simulink model "Demo1_final"  (R2015a)
settings: Solver=ode45  StartTime=0.0  StopTime=inf  RelTol=1e-3
InitFcn:
  | Initilization_simulink
values from neighbouring files (symbols this model uses):
  field_x = sqrt(field_x_vec(1)^2 + field_x_vec(2)^2)    [CalibrateField.m]    (also in Config.mat = 11.7868563762)
  field_y = sqrt(field_y_vec(1)^2 + field_y_vec(2)^2)    [CalibrateField.m]    (also in Config.mat = 8.01974905199)
  items = [CR1;CR2;CR3;CR4]    [CalibrateField.m]    (also in Config.mat = [-6.14339468658  -3.99467558804; 5.6178847579  -4.007837403;)
  ref = [3.07784055213  -4.49067034415  0; -3.25612463225  -4.14482557696  0; 3.15604151052  4.41744641428  0]    [Config.mat]
  thetaCamX = 43*pi/180    (= 0.750491578358)    [Initilization_simulink.m]    (also in debugging_refereeing.m = 1.01229096616)
  thetaCamY = 32*pi/180    (= 0.558505360638)    [Initilization_simulink.m]
undefined symbols (not defined in the file or in its folder): backim, drone1
libraries: visionsinks x2
settings Model: CovSFcnEnable=off  Creator=tzwijger  LastModifiedBy=tzwijger
settings DebuggingCC: SolverPrmCheckMsg=warning

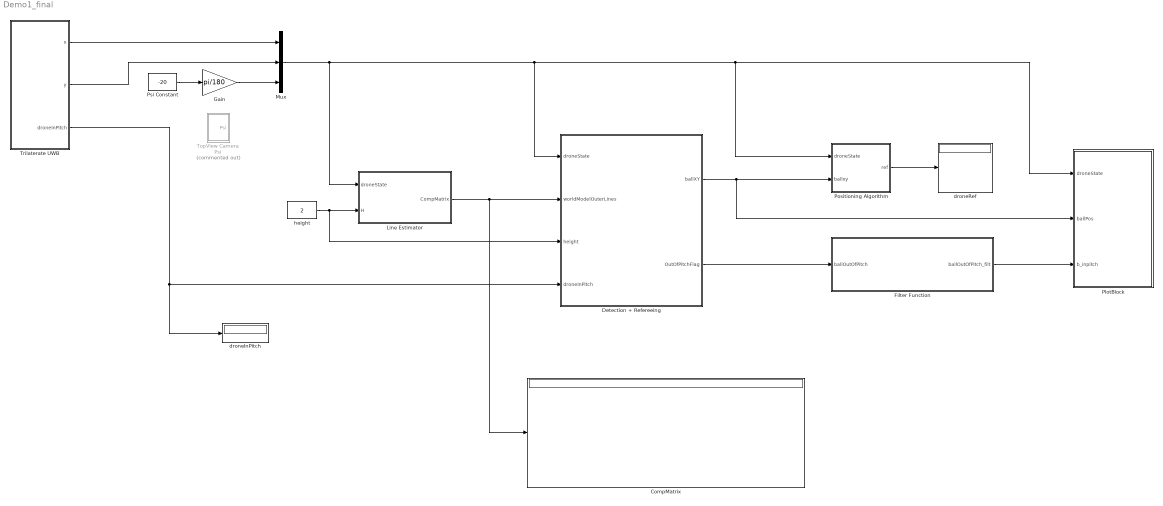
== system Demo1_final ==
  CompMatrix : Display
  Detection + Refereeing : Subsystem
  Filter Function : MATLAB Function  TreatAsAtomicUnit=on
  Gain : Gain  Gain=pi/180
  Line Estimator : Subsystem
  Mux : Mux  Inputs=3
  PlotBlock : Subsystem
  Positioning Algorithm : Subsystem
  Psi Constant : Constant  Value=-20
  TopView Camera Psi : Subsystem  Commented=on
  Trilaterate UWB : Subsystem
  droneInPitch : Display
  droneRef : Display
  height : Constant  Value=2
  wires:
  Line Estimator/1(CompMatrix) -> Detection + Refereeing/2(worldModelOuterLines), CompMatrix/1
  Trilaterate UWB/3(droneInPitch) -> droneInPitch/1, Detection + Refereeing/4(droneInPitch)
  height/1 -> Detection + Refereeing/3(height), Line Estimator/2(H)
  Mux/1 -> Line Estimator/1(droneState), Detection + Refereeing/1(droneState), Positioning Algorithm/1(droneState), PlotBlock/1(droneState)
  Detection + Refereeing/1(ballXY) -> PlotBlock/2(ballPos), Positioning Algorithm/2(ballxy)
  Positioning Algorithm/1(ref) -> droneRef/1
  Trilaterate UWB/1(x) -> Mux/1
  Trilaterate UWB/2(y) -> Mux/2
  Detection + Refereeing/2(OutOfPitchFlag) -> Filter Function/1(ballOutOfPitch)
  Filter Function/1(ballOutOfPitch_filt) -> PlotBlock/3(b_inpitch)
  Psi Constant/1 -> Gain/1
  Gain/1 -> Mux/3

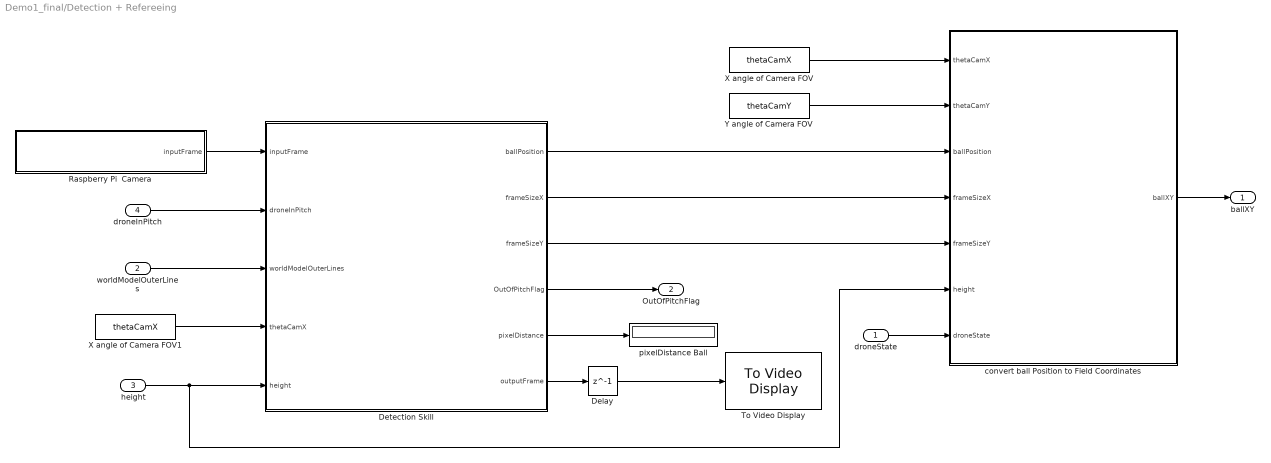
== system Demo1_final/Detection + Refereeing ==
  droneState : Inport
  worldModelOuterLines : Inport  Port=2
  height : Inport  Port=3
  droneInPitch : Inport  Port=4
  Delay : Delay  DelayLength=1  SampleTime=0.25
  Detection Skill : MATLAB Function  TreatAsAtomicUnit=on
  Raspberry Pi  Camera : MATLAB Function  TreatAsAtomicUnit=on
  To Video Display : visionsinks/To Video Display  windowSizeMode=True size (1:1)  openAtMdlStart=on  fullScreen=off  videoWindowX=54  videoWindowY=328  saveWindowSize=off  videoWindowWidth=320  videoWindowHeight=240  inputColorFormat=RGB  inputType=Obsolete  imagePorts=One multidimensional signal  OutputDevice=On-screen video monitor  dataOrg=Column-major  isWindowOpen=off
  X angle of Camera FOV : Constant  Value=thetaCamX
  X angle of Camera FOV1 : Constant  Value=thetaCamX
  Y angle of Camera FOV : Constant  Value=thetaCamY
  convert ball Position to Field Coordinates : Subsystem
  pixelDistance Ball : Display
  ballXY : Outport
  OutOfPitchFlag : Outport  Port=2
  wires:
  droneState/1 -> convert ball Position to Field Coordinates/7(droneState)
  convert ball Position to Field Coordinates/1(ballXY) -> ballXY/1
  X angle of Camera FOV/1 -> convert ball Position to Field Coordinates/1(thetaCamX)
  Y angle of Camera FOV/1 -> convert ball Position to Field Coordinates/2(thetaCamY)
  height/1 -> convert ball Position to Field Coordinates/6(height), Detection Skill/5(height)
  X angle of Camera FOV1/1 -> Detection Skill/4(thetaCamX)
  worldModelOuterLines/1 -> Detection Skill/3(worldModelOuterLines)
  droneInPitch/1 -> Detection Skill/2(droneInPitch)
  Raspberry Pi  Camera/1(inputFrame) -> Detection Skill/1(inputFrame)
  Detection Skill/5(pixelDistance) -> pixelDistance Ball/1
  Detection Skill/4(OutOfPitchFlag) -> OutOfPitchFlag/1
  Detection Skill/1(ballPosition) -> convert ball Position to Field Coordinates/3(ballPosition)
  Detection Skill/2(frameSizeX) -> convert ball Position to Field Coordinates/4(frameSizeX)
  Detection Skill/3(frameSizeY) -> convert ball Position to Field Coordinates/5(frameSizeY)
  Detection Skill/6(outputFrame) -> Delay/1
  Delay/1 -> To Video Display/1

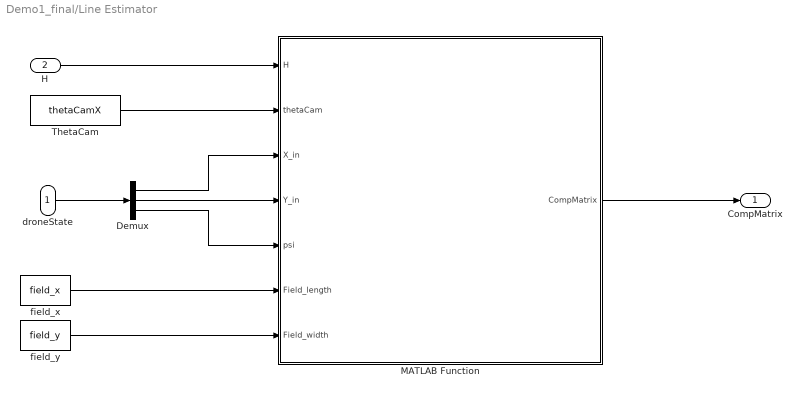
== system Demo1_final/Line Estimator ==
  droneState : Inport
  H : Inport  Port=2
  Demux : Demux  Outputs=3
  MATLAB Function : MATLAB Function  TreatAsAtomicUnit=on
  ThetaCam : Constant  Value=thetaCamX
  field_x : Constant  Value=field_x
  field_y : Constant  Value=field_y
  CompMatrix : Outport
  wires:
  MATLAB Function/1(CompMatrix) -> CompMatrix/1
  ThetaCam/1 -> MATLAB Function/2(thetaCam)
  H/1 -> MATLAB Function/1(H)
  droneState/1 -> Demux/1
  field_x/1 -> MATLAB Function/6(Field_length)
  field_y/1 -> MATLAB Function/7(Field_width)
  Demux/1 -> MATLAB Function/3(X_in)
  Demux/2 -> MATLAB Function/4(Y_in)
  Demux/3 -> MATLAB Function/5(psi)

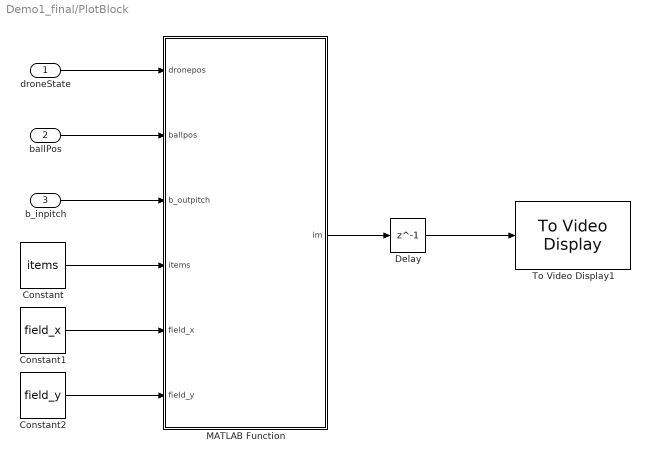
== system Demo1_final/PlotBlock ==
  droneState : Inport
  ballPos : Inport  Port=2
  b_inpitch : Inport  Port=3
  Constant : Constant  Value=items
  Constant1 : Constant  Value=field_x
  Constant2 : Constant  Value=field_y
  Delay : Delay  DelayLength=1  SampleTime=0.25
  MATLAB Function : MATLAB Function  TreatAsAtomicUnit=on
  To Video Display1 : visionsinks/To Video Display  windowSizeMode=True size (1:1)  openAtMdlStart=on  fullScreen=off  videoWindowX=559  videoWindowY=31  saveWindowSize=off  videoWindowWidth=883  videoWindowHeight=607  inputColorFormat=RGB  inputType=Obsolete  imagePorts=One multidimensional signal  OutputDevice=On-screen video monitor  dataOrg=Column-major  isWindowOpen=off
  wires:
  Constant/1 -> MATLAB Function/4(items)
  ballPos/1 -> MATLAB Function/2(ballpos)
  droneState/1 -> MATLAB Function/1(dronepos)
  Constant1/1 -> MATLAB Function/5(field_x)
  Constant2/1 -> MATLAB Function/6(field_y)
  MATLAB Function/1(im) -> Delay/1
  Delay/1 -> To Video Display1/1
  b_inpitch/1 -> MATLAB Function/3(b_outpitch)

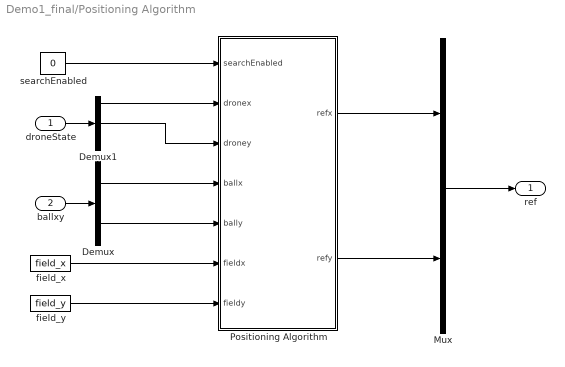
== system Demo1_final/Positioning Algorithm ==
  droneState : Inport
  ballxy : Inport  Port=2
  Demux : Demux  Outputs=2
  Demux1 : Demux  Outputs=3
  Mux : Mux  Inputs=2
  Positioning Algorithm : MATLAB Function  TreatAsAtomicUnit=on
  field_x : Constant  Value=field_x
  field_y : Constant  Value=field_y
  searchEnabled : Constant  Value=0
  ref : Outport
  wires:
  Demux/2 -> Positioning Algorithm/5(bally)
  Demux/1 -> Positioning Algorithm/4(ballx)
  Positioning Algorithm/1(refx) -> Mux/1
  Positioning Algorithm/2(refy) -> Mux/2
  Mux/1 -> ref/1
  field_x/1 -> Positioning Algorithm/6(fieldx)
  field_y/1 -> Positioning Algorithm/7(fieldy)
  droneState/1 -> Demux1/1
  Demux1/1 -> Positioning Algorithm/2(dronex)
  ballxy/1 -> Demux/1
  Demux1/2 -> Positioning Algorithm/3(droney)
  searchEnabled/1 -> Positioning Algorithm/1(searchEnabled)

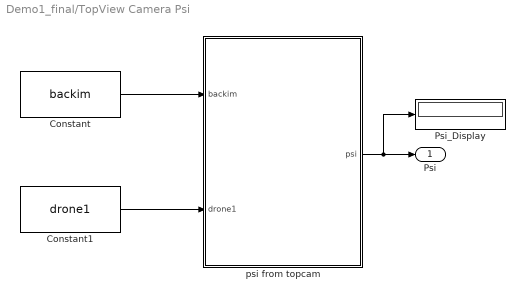
== system Demo1_final/TopView Camera Psi ==
  Constant : Constant  Value=backim
  Constant1 : Constant  Value=drone1
  Psi_Display : Display
  psi from topcam : MATLAB Function  TreatAsAtomicUnit=on
  Psi : Outport
  wires:
  Constant1/1 -> psi from topcam/2(drone1)
  Constant/1 -> psi from topcam/1(backim)
  psi from topcam/1(psi) -> Psi_Display/1, Psi/1

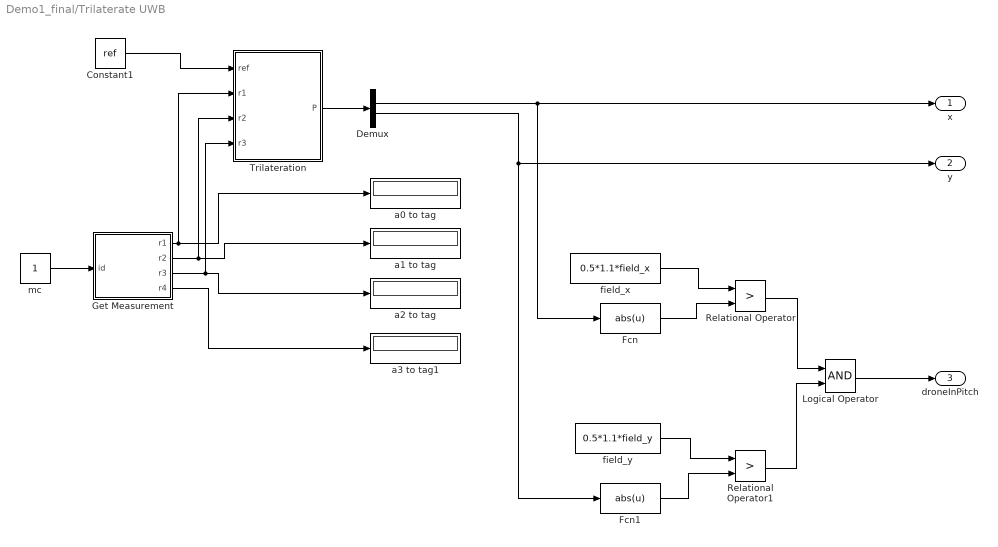
== system Demo1_final/Trilaterate UWB ==
  Constant1 : Constant  Value=ref
  Demux : Demux
  Fcn : Fcn  Expr=abs(u)
  Fcn1 : Fcn  Expr=abs(u)
  Get Measurement : MATLAB Function  TreatAsAtomicUnit=on
  Logical Operator : Logic  AllPortsSameDT=off  OutDataTypeStr=boolean
  Relational Operator : RelationalOperator  Operator=>  OutDataTypeStr=boolean
  Relational Operator1 : RelationalOperator  Operator=>  OutDataTypeStr=boolean
  Trilateration : MATLAB Function  TreatAsAtomicUnit=on
  a0 to tag : Display
  a1 to tag : Display
  a2 to tag : Display
  a3 to tag1 : Display
  field_x : Constant  Value=0.5*1.1*field_x
  field_y : Constant  Value=0.5*1.1*field_y
  mc : Constant
  x : Outport
  y : Outport  Port=2
  droneInPitch : Outport  Port=3
  wires:
  Demux/3 -> Fcn1/1, y/1
  Demux/2 -> Fcn/1, x/1
  Trilateration/1(P) -> Demux/1
  Constant1/1 -> Trilateration/1(ref)
  Get Measurement/3(r3) -> a2 to tag/1, Trilateration/4(r3)
  Get Measurement/2(r2) -> a1 to tag/1, Trilateration/3(r2)
  mc/1 -> Get Measurement/1(id)
  Get Measurement/1(r1) -> Trilateration/2(r1), a0 to tag/1
  Get Measurement/4(r4) -> a3 to tag1/1
  Fcn/1 -> Relational Operator/2
  field_x/1 -> Relational Operator/1
  field_y/1 -> Relational Operator1/1
  Fcn1/1 -> Relational Operator1/2
  Relational Operator1/1 -> Logical Operator/2
  Relational Operator/1 -> Logical Operator/1
  Logical Operator/1 -> droneInPitch/1

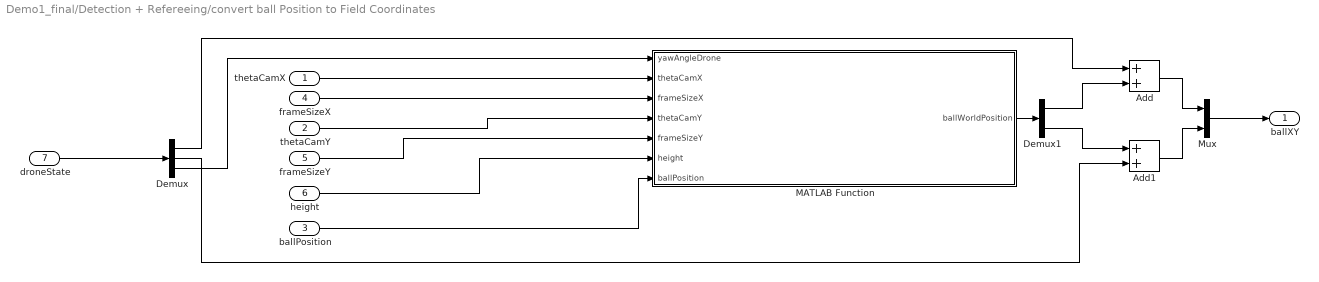
== system Demo1_final/Detection + Refereeing/convert ball Position to Field Coordinates ==
  thetaCamX : Inport
  thetaCamY : Inport  Port=2
  ballPosition : Inport  Port=3
  frameSizeX : Inport  Port=4
  frameSizeY : Inport  Port=5
  height : Inport  Port=6
  droneState : Inport  Port=7
  Add : Sum
  Add1 : Sum
  Demux : Demux  Outputs=3
  Demux1 : Demux  Outputs=2
  MATLAB Function : MATLAB Function  TreatAsAtomicUnit=on
  Mux : Mux  Inputs=2
  ballXY : Outport
  wires:
  thetaCamY/1 -> MATLAB Function/4(thetaCamY)
  height/1 -> MATLAB Function/6(height)
  thetaCamX/1 -> MATLAB Function/2(thetaCamX)
  ballPosition/1 -> MATLAB Function/7(ballPosition)
  frameSizeY/1 -> MATLAB Function/5(frameSizeY)
  Mux/1 -> ballXY/1
  Add/1 -> Mux/1
  Add1/1 -> Mux/2
  MATLAB Function/1(ballWorldPosition) -> Demux1/1
  frameSizeX/1 -> MATLAB Function/3(frameSizeX)
  Demux/1 -> Add/1
  Demux1/2 -> Add1/1
  Demux1/1 -> Add/2
  droneState/1 -> Demux/1
  Demux/3 -> MATLAB Function/1(yawAngleDrone)
  Demux/2 -> Add1/2

== matlab function Demo1_final/Trilaterate UWB/Trilateration ==
  data: P output; ref input; r1 input; r2 input; r3 input
function P  = trilateration(ref,r1,r2,r3)%,fign,field2im_params)
% persistent plots k nrplots

coder.extrinsic('Trilateration')

% if isempty(plots)
%     plots = [0];
%     k = 1;
%     nrplots = 10;
% end

P = zeros(4,1);
P = Trilateration(ref',[r1 r2 r3],eye(3));

% % Plot and print results
% [plots, k] = update_plot_trilat(plots, k, fign, P(2:3), field2im_params, nrplots);

== matlab function Demo1_final/Trilaterate UWB/Get Measurement ==
  data: id input; r1 output; r2 output; r3 output; r4 output
function [r1,r2,r3,r4] = GetMC_sm(id) 
    % Input: Serial Port to A0
    %        
    % Output: Raw data for triangulation
    %
    % Message syntax is explained in the Decawave documentation
    % DecaRangeRTLS_PC_Source_Code_Guide.pdf  - Section 2.3.2
    % DecaRangeRTLS_ARM_Source_Code_Guide.pdf - Section 2.6

    % Make sure to get a measurement with the correct identifier
    persistent s count;
    %coder.extrinsic('instrfind','delete','serial','fscanf','strsplit')
    coder.extrinsic('instrfind','delete','serial','fscanf','GetMC','flushinput')
    
    r1 = 0; r2 = 0; r3 = 0; r4 = 0;
    
    if isempty(s)
        ports = instrfind;
        if ~isempty(ports)
            fclose(ports);
            delete(ports);
        end
        % Establish new connection
        s = serial('COM33','BaudRate',9600,'Parity','None');

        % Open connection
        fopen(s);
        fscanf(s); % Get init mc out of the way and test connection
        
        count = 0;
    end
    
    ids = ['mc';'mr';'ma'];
    id = ids(id,:);
    
    dist = zeros(1,4);
    
    dist = GetMC(s,id);
    r1 = dist(1);
    r2 = dist(2);
    r3 = dist(3);
    r4 = dist(4); 
    
    if count > 10
        % We are reading values slower than they come in
        % Sometimes the buffer needs to be cleared
        flushinput(s)
        count = 0;
    else
        count = count + 1;
    end
end

== matlab function Demo1_final/Line Estimator/MATLAB Function ==
  data: H input; CompMatrix output; thetaCam input; X_in input; Y_in input; psi input; Field_length input; Field_width input
function CompMatrix   = World(H,thetaCam,X_in,Y_in,psi,Field_length,Field_width)

% %field line numbering:  222222222222222222223
%                         1                   3
%                         1                   3
%                         1                   3
%                         1                   3
%                         1                   3
%                         144444444444444444443

% Psi: conter-clock wise positive. zero at localization Y axis
% Theta and rho are defined according to matlab hough transform matrix

Vision=2*H*tan(thetaCam/2);

X_Vision=Vision;  %<--------------->
% Y_Vision=Vision*(480/640);  %|
                            %|

% Lvision=sqrt((X_Vision^2)+(Y_Vision^2));
% init_angel=atan(640/480);
% X=X_in-(Lvision/2)*sin(init_angel-psi);  %moving the origin from center of the camera to top left
% Y=Y_in+(Lvision/2)*cos(init_angel-psi);
%%%%%%%%%%%%%%%%%%%%%%%%%%%%%%%%%%%%%%%%%%%%%%%%%%%%%%%%%%%%%%%%%%%%%%%%%%
%Field_length=10;   %dimentions of the field%<--------------->

%Field_width=8; %|
                %|

pixelDistanceWorld=(H*tan(thetaCam/2))/(320/2);
Rx2=rotx(-180);
Rz2=rotz(psi*180/pi);
P2=[-320/2*pixelDistanceWorld;-240/2*pixelDistanceWorld; 0];
P3=Rx2*Rz2*P2;
P4=[X_in+P3(1) Y_in+P3(2)];
                
%%%%%%%%%%%%%%%%%%%%%%%%%%%%%%%%%%%%%%%%%%%%%%%%%%%%%%%%%%%%%%%%%%%%%%%%%%%
rho1=abs(P4(1)+(Field_length)/2); %calculate rho of each side line with respect to top left cordinate
rho2=abs(-P4(2)+(Field_width)/2);
rho3= abs(-P4(1)+(Field_length)/2);
rho4= abs(P4(2)+(Field_width)/2);
%%%%%%%%%%%%%%%%%%%%%%%%%%%%%%%%%%%%%%%%%%%%%%%%%%%%%%%%%%%%%%%%%%%%%%%%
X1=X_in;  %having center to compare the distance and rho
Y1=Y_in;

rho11=abs(X1+(Field_length)/2);
rho21=abs(-Y1+(Field_width)/2);
rho31= abs(-X1+(Field_length)/2);
rho41= abs(Y1+(Field_width)/2);



%%%%%%%%%%%%%%%%%%%%%%%%%%%%%%%%%%%%%%%%%%%%%%%%%%%%%%%%%%%%%%%%%%%%%%%%%%
theta1=(pi)-psi;       %calculate the theta of each side line
theta2=(-pi/2)-psi;
theta3=(0)-psi;
theta4=(pi/2)-psi;
%%%%%%%%%%%%%%%%%%%%%%%%%%%%%%%%%%%%%%%%%%%%%%%%%%%%%%%%%%%%%%%%%%%%%%%%%%

Lines=[rho1,theta1,rho11;
rho2,theta2,rho21;
rho3,theta3,rho31;
rho4,theta4,rho41];
B=zeros(4,5);



for k=1:4
    
    i=0;
    rho=Lines(k,1);
    theta=Lines(k,2);
    %if -Y_Vision*sin(theta)<rho &&  rho<X_Vision*cos(theta)
    if Lines(k,3)<X_Vision/2
        i=1;
        

    end
    while theta>=(2*pi) 
        theta=theta-2*pi;
    end
    while theta<0
        theta=theta+2*pi;
    end
    
        while theta>=(pi/2) 
        theta=theta-pi;
    end
    while theta<-pi/2
        theta=theta+pi;
    end
    
    B(k,:)=[k i 0 rho theta];
end
B(1,3)=2;
B(2,3)=1;
B(3,3)=2;
B(4,3)=1;

CompMatrix=zeros(4,5);
CompMatrix=B;

== matlab function Demo1_final/Detection + Refereeing/Detection Skill ==
  data: inputFrame input; droneInPitch input; worldModelOuterLines input; thetaCamX input; height input; ballPosition output; frameSizeX output; frameSizeY output; OutOfPitchFlag output; pixelDistance output; outputFrame output
% Author: Nestor Hernandez Rodriguez
% Last Update: 9-03-2016
% Technical University of Eindhoven
% Mechatronic Systems Design PDEng trainee

function [ballPosition,...
          frameSizeX,...
          frameSizeY,...
          OutOfPitchFlag,...
          pixelDistance,...
          outputFrame] = detectionSkillAndRefereeing(...
                                                    inputFrame,...
                                                    droneInPitch,...
                                                    worldModelOuterLines,...
                                                    thetaCamX,...
                                                    height)
                                                 
    coder.extrinsic('detectionSkill','refereeingOutOfPitch','imresize')
    
    % Prepare outputs detection skill
    ballPosition = zeros(1,2);
    %selectedLines = zeros(50,2);
    ballStatusFlag = 0;
    lineStatusFlag = 0;
    %inputFrame = imresize(inputFrame,0.65,'bilinear');
    
    outputFrame = uint8(zeros(size(inputFrame)));
    
    % Prepare outputs Refereeing function
    OutOfPitchFlag = 0;
%     selectedFilteredLines = zeros(2,6);
    pixelDistance=0;
    
    % Prepare constant/unused inputs Refereeing function
    numOutOfBoundLines = 0;
    numOutOfBoundLines = sum(worldModelOuterLines(:,2));
    
    % Prepare Other Inputs
    temp = size(inputFrame);
    frameSizeX = temp(2);
    frameSizeY = temp(1);
    frameProperties = [frameSizeY frameSizeX];
    if sum(worldModelOuterLines(:,2)) > 0
        lineDetectionEnabled = 1;
    else
        lineDetectionEnabled = 0; 
    end
    
    [ballPosition,... 
     selectedLines,... 
     outputFrame] = detectionSkill(lineDetectionEnabled,...
                                   inputFrame);
                               
    selectedLines                                                             
    [OutOfPitchFlag,...
        pixelDistance]= refereeingOutOfPitch(...
                                           ballPosition,...
                                           selectedLines,...
                                           numOutOfBoundLines,...
                                           frameProperties,...
                                           droneInPitch,...
                                           thetaCamX,...
                                           height,...                                           
                                           worldModelOuterLines);
end

== matlab function Demo1_final/TopView Camera Psi/psi from topcam ==
  data: backim input; psi output; drone1 input
function psi = fcn(backim, drone1)
%% get psi angle from top camera
% this function is the improcdrones.m implemented for ONLY ONE DRONE and 
% therefore reduced.




coder.extrinsic('psi_topviewcam_wrapped')
    
    psi = 0;
    psi = psi_topviewcam_wrapped(backim, drone1);

end

== matlab function Demo1_final/Positioning Algorithm/Positioning Algorithm ==
  data: searchEnabled input; dronex input; droney input; ballx input; refx output; bally input; refy output; fieldx input; fieldy input
function [refx,refy] = positionDrone(searchEnabled,dronex,droney,ballx,bally,fieldx,fieldy)
% ball position [-999 -999] -> No Ball Position Known
    persistent searchArray count step
    if isempty(searchArray)
       count = 1;
       i = 1;
       step = 1;
       searchArray = zeros(100,2);% Size HAS to be predetermined (...Simulink...)
       for y = -0.5*fieldy:step:0.5*fieldy
          searchArray(i,:) =  [-0.5*fieldx,y];
          searchArray(i+1,:) =  [0.5*fieldx,y];
          i = i + 2;
       end
    end
    refx = 0;
    refy = 0;

    if ballx ~= -999 && bally ~= -999
        % Ball Position is known
        if abs(ballx) < 0.5*fieldx && abs(bally) < 0.5*fieldy
            % Ball is in field
            refx = ballx; 
            refy = bally;
        else
            % Ball is out of field
            % Go as close as possible without leaving the field
            refx = sign(ballx)*min(abs(ballx),0.5*fieldx);
            refy = sign(bally)*min(abs(bally),0.5*fieldy);       
        end
        % Reset count if search was enabled
        if count ~= 1
            count = 1;
        end
    elseif searchEnabled
        % Ball position is not known, search sequence initiated
        if (abs(dronex) - searchArray(count,1) < 0.25 ||...
            abs(droney) - searchArray(count,2) < 0.25)
            if count < 2*floor(fieldy/step)
                count = count + 1;
            else
                count = 1;
            end
        end
        refx = searchArray(count,1);
        refy = searchArray(count,2);
    else
        % Search disabled, hover over origin
        refx = 0;
        refy = 0;
    end

== matlab function Demo1_final/Detection + Refereeing/convert ball Position to Field Coordinates/MATLAB Function ==
  data: yawAngleDrone input; thetaCamX input; frameSizeX input; thetaCamY input; frameSizeY input; height input; ballPosition input; ballWorldPosition output
% Author: Nestor Hernandez Rodriguez
% Last Update: 15-03-2016
% Technical University of Eindhoven
% Mechatronic Systems Design PDEng trainee

function ballWorldPosition =frameToWorldCoordinates(yawAngleDrone, thetaCamX, frameSizeX, thetaCamY, frameSizeY, height, ballPosition)

% This function carries out the ball position conversion from pixel frame
% coordinates to world model coordinates in meters
% 
% Inputs:
% ballPosition - 2x1 vector containing the center of the ball in the frame
%
% yawAngleDrone - yaw angle of the drone referenced to the world model coordinate system in radians
%
% thetaCamX, thetaCamY - angle in radians of the FOV of the camera used for both axis
%
% frameSizeX, frameSizeY - resolution in pixels for both axis
% 
% height - height of the drone in meters
%
% Outputs:
% ballWorldPosition - 2x1 vector containing the center of the ball in the
% frame referenced to the world model coordinate system orientation in
% meters



% Calculate Rotation matrix between the frame reference system and the
% world reference system
if ballPosition(1) == -100 && ballPosition(2) == -100
    ballWorldPosition = [-999 -999];
else    
    %syms t;

    %x_Rot = [1 0 0; 0 cos(t) -sin(t); 0 sin(t) cos(t)];
    %z_Rot = [cos(t) -sin(t) 0; sin(t) cos(t) 0; 0 0 1];

    Rx=rotx(-180);%eval(subs(x_Rot, t, -pi));
    Rz=rotz(yawAngleDrone*180/pi);%eval(subs(z_Rot, t, yawAngleDrone));


    % Calculate ball position with respect to the center of the frame

    ballPosition2=[ballPosition(1)-frameSizeX/2; ballPosition(2)-frameSizeY/2; 0];

    % Calculate vector in the local reference system with the same orientation
    % as the absolute reference system

    ballPosition3=Rx*Rz*ballPosition2;

    % Translate pixel distance into meters for both axis (Using two thetas is
    % more accurate)

    pixelDistanceX = (height*tan(thetaCamX/2))/(frameSizeX/2);
    pixelDistanceY = (height*tan(thetaCamY/2))/(frameSizeY/2);

    % Calculating ball position in meters

    ballWorldPosition=[ballPosition3(1)*pixelDistanceX ballPosition3(2)*pixelDistanceY];
end

== matlab function Demo1_final/Detection + Refereeing/Raspberry Pi  Camera ==
  data: inputFrame output
function inputFrame = rasPiCam()    	
    coder.extrinsic('getFramePi')

    inputFrame = uint8(zeros(240,320,3));
    inputFrame = getFramePi();
end

== matlab function Demo1_final/PlotBlock/MATLAB Function ==
  data: dronepos input; im output; ballpos input; b_outpitch input; items input; field_x input; field_y input
function im  = update_plot_trilat(dronepos, ballpos, b_outpitch, items, field_x, field_y)
    
    persistent im_init field2im_params
    
    coder.extrinsic('init_plot_trilat_img','update_plot_trilat_img')    
        
    if (isempty(im_init)||isempty(field2im_params))
        [im_init,field2im_params] = init_plot_trilat_img(items,field_x,field_y);        
    end
    
    %im = uint8(zeros(542,810,3));
    im = uint8(zeros(607,883,3));
    im = update_plot_trilat_img(im_init,field2im_params,ballpos,dronepos,b_outpitch);   
end

== matlab function Demo1_final/Filter Function ==
  data: ballOutOfPitch input; ballOutOfPitch_filt output
function ballOutOfPitch_filt  = filter(ballOutOfPitch)
    persistent pastVals
    
    numPastVals = 10;
    
    if isempty(pastVals)
       pastVals = -1*ones(numPastVals,1);
    end
    
    pastVals = [ballOutOfPitch; pastVals(1:numPastVals-1)];      
    
    if length(pastVals == -1) > max([length(pastVals == 0);length(pastVals == 1)])
        ballOutOfPitch_filt = -1;
    else
        pastVals_mean = mean(pastVals(pastVals ~= -1));
        if pastVals_mean > 0.55
            ballOutOfPitch_filt = 1;
        elseif pastVals_mean < 0.45
            ballOutOfPitch_filt = 0;
        else
            ballOutOfPitch_filt = -1;
        end
    end
